simulink model "scheme_1"  (R2023a)
settings: Solver=VariableStepAuto  StartTime=0.0  StopTime=10  RelTol=1e-8
settings Model: Creator=user  LastModifiedBy=user

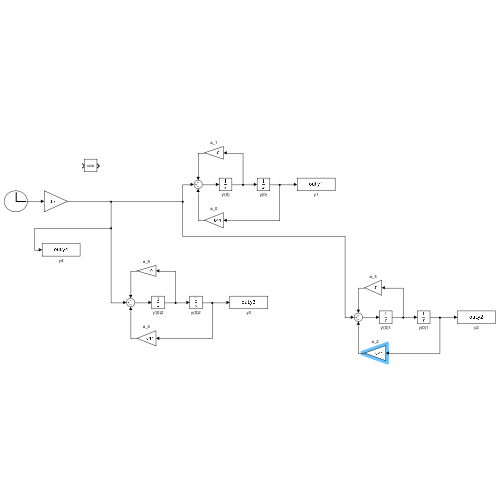
[thumbnail: Simulink's stored preview of the top-level diagram]
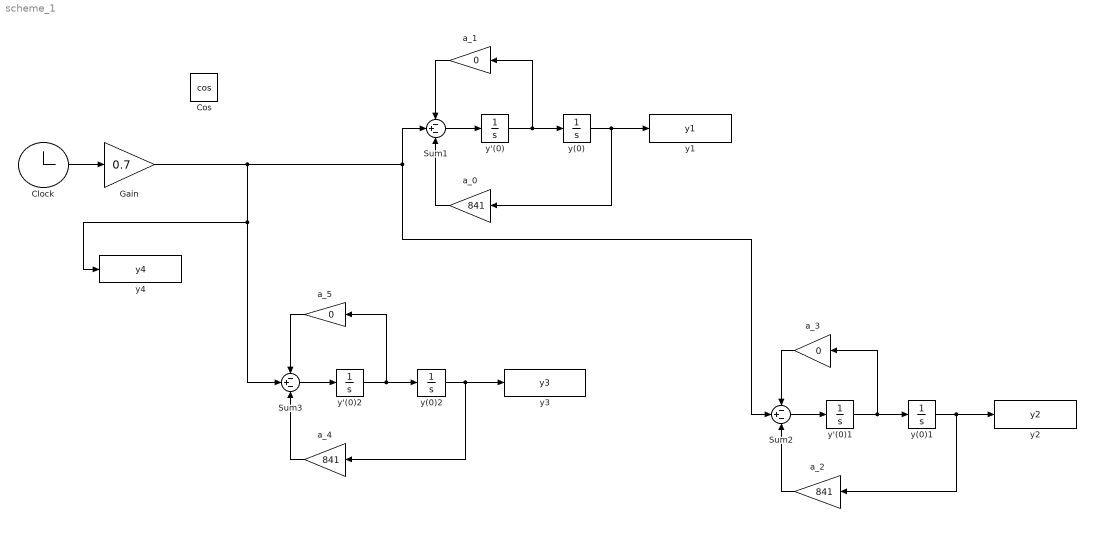
== system scheme_1 ==
  Clock : Clock
  Cos : Trigonometry  Operator=cos
  Gain : Gain  Gain=0.7
  Sum1 : Sum  Inputs=-+-
  Sum2 : Sum  Inputs=-+-
  Sum3 : Sum  Inputs=-+-
  a_0 : Gain  Gain=841
  a_1 : Gain  Gain=0
  a_2 : Gain  Gain=841
  a_3 : Gain  Gain=0
  a_4 : Gain  Gain=841
  a_5 : Gain  Gain=0
  y'(0) : Integrator
  y'(0)1 : Integrator
  y'(0)2 : Integrator
  y(0) : Integrator  InitialCondition=-1
  y(0)1 : Integrator
  y(0)2 : Integrator  InitialCondition=1
  y1 : ToWorkspace  VariableName=y1  SaveFormat=Timeseries  SampleTime=-1
  y2 : ToWorkspace  VariableName=y2  SaveFormat=Timeseries  SampleTime=-1
  y3 : ToWorkspace  VariableName=y3  SaveFormat=Timeseries  SampleTime=-1
  y4 : ToWorkspace  VariableName=y4  SaveFormat=Timeseries  SampleTime=-1
  wires:
  a_0/1 -> Sum1/3
  a_1/1 -> Sum1/1
  Sum1/1 -> y'(0)/1
  y'(0)/1 -> a_1/1, y(0)/1
  y(0)/1 -> a_0/1, y1/1
  a_2/1 -> Sum2/3
  a_3/1 -> Sum2/1
  Sum2/1 -> y'(0)1/1
  y'(0)1/1 -> a_3/1, y(0)1/1
  y(0)1/1 -> a_2/1, y2/1
  a_4/1 -> Sum3/3
  a_5/1 -> Sum3/1
  Sum3/1 -> y'(0)2/1
  y'(0)2/1 -> a_5/1, y(0)2/1
  y(0)2/1 -> a_4/1, y3/1
  Clock/1 -> Gain/1
  Gain/1 -> y4/1, Sum3/2, Sum2/2, Sum1/2
